simulink model "ElectronicStabilityControl"  (R2025b)
settings: configuration reference "VehicleFixed10ms" (kept outside this file)
undefined symbols (not defined in the file): CtrlBcuTrlrBrkGain, PlntVehDstCGFrntAxl, PlntVehDstCGRearAxl, vehdynicon
libraries: slpidlib x1, simulink x1
settings Model: DataDictionary=VirtualVehicleTemplate.sldd  ModifiedByFormat=The MathWorks, Inc.  Creator=The MathWorks, Inc.  LastModifiedBy=The MathWorks, Inc.
settings ConfigSetRef: SourceName=VehicleFixed10ms

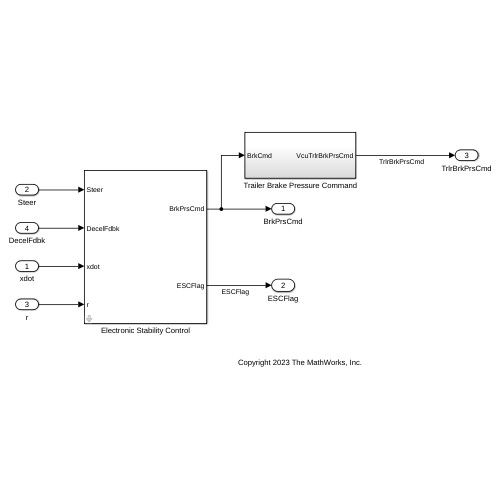
[thumbnail: Simulink's stored preview of the top-level diagram]
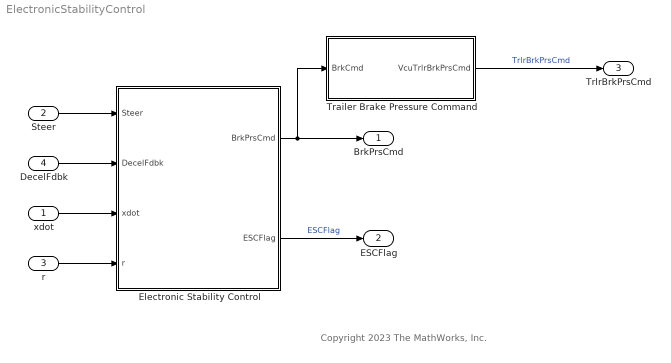
== system ElectronicStabilityControl ==
  note: Copyright 2023 The MathWorks, Inc.
  xdot : Inport  OutDataTypeStr=double  PortDimensions=1
  Steer : Inport  Port=2  OutDataTypeStr=double  PortDimensions=1
  r : Inport  Port=3  OutDataTypeStr=double  PortDimensions=1
  DecelFdbk : Inport  Port=4  OutDataTypeStr=double  PortDimensions=1
  Electronic Stability Control : Subsystem  mask{USG=1.15, xdot_en=2, L=PlntVehDstCGFrntAxl + PlntVehDstCGRearAxl, g=9.8, mu=1, xdotbpt=[-60:10:60], PGain=[.1 .2 .5 .8 1.5 3.0 0 3.0 1.5 .8 .5 .2 .1]}
      mask prompts: USG "Understeering gradient, USG [deg/g]:"; xdot_en "Speed threshold of ESC activation, xdot_en [m/s]:"; L "Wheel base, L [m]:"; g "Gravity acceleration, g [m/s^2]:"; mu "Tire-road scaling friction coefficient, mu []:"; xdotbpt "Speed breakpoints, xdotbpt [m/s]:"; PGain "P gain table data, PGain []:"
      mask help: This block offers Electronic Stability Control (ESC), a system designed to uphold a vehicle lateral and yaw stability by autonomously modulating brake pressure.
      mask init:
      | vehdynicon('vehdynalgo', gcb);
      mask DialogControl Container4 Prompt: Constants
      mask DialogControl Container3 Prompt: Controller parameters
  Trailer Brake Pressure Command : Subsystem
  BrkPrsCmd : Outport  OutDataTypeStr=double  VectorParamsAs1DForOutWhenUnconnected=off
  ESCFlag : Outport  Port=2  OutDataTypeStr=boolean
  TrlrBrkPrsCmd : Outport  Port=3  PortDimensions=6  VectorParamsAs1DForOutWhenUnconnected=off
  wires:
  Trailer Brake Pressure Command/1(VcuTrlrBrkPrsCmd) -> TrlrBrkPrsCmd/1  "TrlrBrkPrsCmd"
  Electronic Stability Control/1(BrkPrsCmd) -> Trailer Brake Pressure Command/1(BrkCmd), BrkPrsCmd/1
  Electronic Stability Control/2(ESCFlag) -> ESCFlag/1  "ESCFlag"
  xdot/1 -> Electronic Stability Control/3(xdot)
  r/1 -> Electronic Stability Control/4(r)
  DecelFdbk/1 -> Electronic Stability Control/2(DecelFdbk)
  Steer/1 -> Electronic Stability Control/1(Steer)

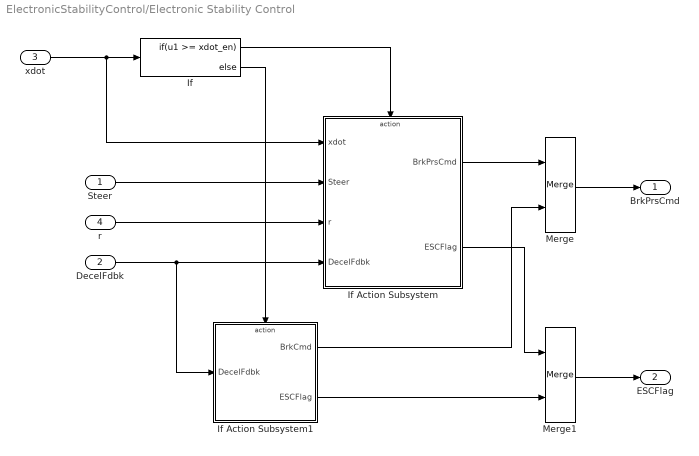
== system ElectronicStabilityControl/Electronic Stability Control ==
  Steer : Inport
  DecelFdbk : Inport  Port=2
  xdot : Inport  Port=3
  r : Inport  Port=4
  If : If  IfExpression=u1 >= xdot_en
  If Action Subsystem : Subsystem  TreatAsAtomicUnit=on
  If Action Subsystem1 : Subsystem  TreatAsAtomicUnit=on
  Merge : Merge
  Merge1 : Merge
  BrkPrsCmd : Outport
  ESCFlag : Outport  Port=2
  wires:
  xdot/1 -> If Action Subsystem/1(xdot), If/1
  Steer/1 -> If Action Subsystem/2(Steer)
  r/1 -> If Action Subsystem/3(r)
  Merge/1 -> BrkPrsCmd/1
  Merge1/1 -> ESCFlag/1
  If/1 -> If Action Subsystem/Action
  DecelFdbk/1 -> If Action Subsystem1/1(DecelFdbk), If Action Subsystem/4(DecelFdbk)
  If/2 -> If Action Subsystem1/Action
  If Action Subsystem1/1(BrkCmd) -> Merge/2
  If Action Subsystem1/2(ESCFlag) -> Merge1/2
  If Action Subsystem/2(ESCFlag) -> Merge1/1
  If Action Subsystem/1(BrkPrsCmd) -> Merge/1

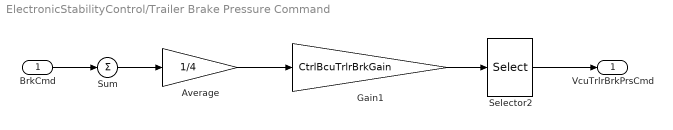
== system ElectronicStabilityControl/Trailer Brake Pressure Command ==
  BrkCmd : Inport
  Average : Gain  Gain=1/4
  Gain1 : Gain  Gain=CtrlBcuTrlrBrkGain
  Selector2 : Selector  InputPortWidth=1  IndexOptions=Index vector (dialog)  Indices=[1 1 1 1 1 1]  OutputSizes=1
  Sum : Sum  Inputs=+
  VcuTrlrBrkPrsCmd : Outport
  wires:
  Gain1/1 -> Selector2/1
  Average/1 -> Gain1/1
  BrkCmd/1 -> Sum/1
  Sum/1 -> Average/1
  Selector2/1 -> VcuTrlrBrkPrsCmd/1

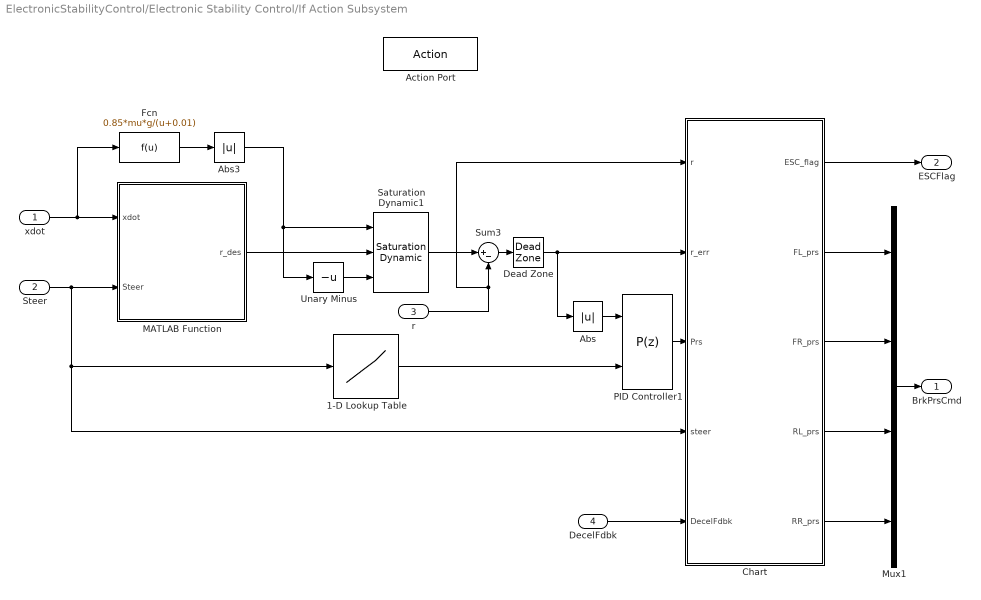
== system ElectronicStabilityControl/Electronic Stability Control/If Action Subsystem ==
  xdot : Inport
  Steer : Inport  Port=2
  r : Inport  Port=3
  DecelFdbk : Inport  Port=4
  Action Port : ActionPort
  1-D Lookup Table : Lookup_n-D  NumberOfTableDimensions=1  BreakpointsForDimension1=xdotbpt  Table=PGain  InternalRulePriority=Speed  RndMeth=Simplest
  Abs : Abs  SaturateOnIntegerOverflow=off
  Abs3 : Abs  SaturateOnIntegerOverflow=off
  Chart : Stateflow chart  InitFcn=vehdynicon('vehdynalgo', gcb);  TreatAsAtomicUnit=on
  Dead Zone : DeadZone  LowerValue=-0.001  UpperValue=0.001
  Fcn : Fcn  Expr=0.85*mu*g/(u+0.01)
  MATLAB Function : MATLAB Function  InitFcn=vehdynicon('vehdynalgo', gcb);  TreatAsAtomicUnit=on
  Mux1 : Mux
  PID Controller1 : slpidlib/PID Controller  Controller=P  Form=Parallel  TimeDomain=Discrete-time  UseExternalTs=off  SampleTime=-1  IntegratorMethod=Forward Euler  FilterMethod=Forward Euler  ControllerParametersSource=external  P=1  I=1  UseKiTs=off  D=0  UseExternalDerivativeSource=off  N=100  UseFilter=on  TunerSelectOption=Transfer Function Based (PID Tuner App)  ZeroCross=off  InitialConditionSource=internal  InitialConditionForIntegrator=0  InitialConditionForFilter=0  DifferentiatorICPrevScaledInput=0  ExternalReset=none  TrackingMode=off  Kt=1  LimitOutput=on  SatLimitsSource=internal  UpperSaturationLimit=1  LowerSaturationLimit=0  LinearizeAsGain=on  AntiWindupMode=none  Kb=1  LimitIntegrator=off  UpperIntegratorSaturationLimit=inf  LowerIntegratorSaturationLimit=-inf  POutMin=[]  POutMax=[]  IOutMin=[]  IOutMax=[]  DOutMin=[]  DOutMax=[]  NOutMin=[]  NOutMax=[]  SumOutMin=[]  SumOutMax=[]  SaturationOutMin=[]  SaturationOutMax=[]  PParamMin=[]  PParamMax=[]  IParamMin=[]  IParamMax=[]  DParamMin=[]  DParamMax=[]  NParamMin=[]  NParamMax=[]  KbParamMin=[]  KbParamMax=[]  KtParamMin=[]  KtParamMax=[]  KbOutMin=[]  KbOutMax=[]  KtOutMin=[]  KtOutMax=[]  IntegratorOutMin=[]  IntegratorOutMax=[]  FilterOutMin=[]  FilterOutMax=[]  SumI1OutMin=[]  SumI1OutMax=[]  SumI2OutMin=[]  SumI2OutMax=[]  SumI3OutMin=[]  SumI3OutMax=[]  SumI4OutMin=[]  SumI4OutMax=[]  SumDOutMin=[]  SumDOutMax=[]  DifferentiatorOutMin=[]  DifferentiatorOutMax=[]  FilterDiffOutCoefMin=[]  FilterDiffOutCoefMax=[]  ReciprocalOutMin=[]  ReciprocalOutMax=[]  SumDenOutMin=[]  SumDenOutMax=[]  SumNumOutMin=[]  SumNumOutMax=[]  DivideOutMin=[]  DivideOutMax=[]  UdiffTsProdOutMin=[]  UdiffTsProdOutMax=[]  NTsProdOutMin=[]  NTsProdOutMax=[]  UintegralTsProdOutMin=[]  UintegralTsProdOutMax=[]  UngainTsProdOutMin=[]  UngainTsProdOutMax=[]  ClampingZeroOutDataTypeStr=Inherit: Inherit via back propagation  ClampingZeroOutMin=[]  ClampingZeroOutMax=[]  FilterDenConstantOutDataTypeStr=Inherit: Inherit via back propagation  FilterDenConstantOutMin=[]  FilterDenConstantOutMax=[]  PCopyOutDataTypeStr=Inherit: Inherit via back propagation  PCopyOutMin=[]  PCopyOutMax=[]  NCopyOutDataTypeStr=Inherit: Inherit via back propagation  NCopyOutMin=[]  NCopyOutMax=[]  IntegratorContinuousStateAttributes=''  IntegratorStateMustResolveToSignalObject=off  IntegratorRTWStateStorageClass=Auto  FilterContinuousStateAttributes=''  FilterStateMustResolveToSignalObject=off  FilterRTWStateStorageClass=Auto  ParallelPVariant=ExternalParameters  IdealPVariant=Disabled  IVariant=Disabled  DVariant=Disabled  IntegratorVariant=Disabled  SatVariant=Enabled  AWVariant=Disabled  PCopyVariant=Disabled  TRVariant=Disabled  FdbkBlocksVariant=Forward  IdealPFdbkVariant=Disabled  SatFdbkVariant=Disabled  DerivativeFilterVariant=Disabled  NVariant=Disabled  NCopyVariant=Disabled_SignalSpec  FilterICVariant=Disabled  IntegratorICVariant=Disabled  ExternalResetVariant=Disabled  TRSumVariant=Passthrough  SumFdbkVariant=Disabled  SumVariant=Passthrough_P  TsampFilterVariant=InternalTs  TsampNgainVariant=Passthrough  TsampIntegralVariant=Disabled_SignalSpec  ExternalSaturationOutDataTypeStr=Inherit: Same as second input  DerivativeSourceVariant=Disabled  PreIntVariant=InternalPreInt
  Saturation Dynamic1 : simulink/Discontinuities/Saturation Dynamic  OutMin=[]  OutMax=[]  OutDataTypeStr=Inherit: Same as second input  OutDataType=fixdt(1, 16)  OutScaling=2^-10  DoSatur=off
  Sum3 : Sum  Inputs=|+-
  Unary Minus : UnaryMinus
  BrkPrsCmd : Outport
  ESCFlag : Outport  Port=2
  wires:
  MATLAB Function/1(r_des) -> Saturation Dynamic1/2
  Chart/4(RL_prs) -> Mux1/3
  Fcn/1 -> Abs3/1
  Mux1/1 -> BrkPrsCmd/1
  Unary Minus/1 -> Saturation Dynamic1/3
  Chart/1(ESC_flag) -> ESCFlag/1
  Chart/3(FR_prs) -> Mux1/2
  Chart/2(FL_prs) -> Mux1/1
  xdot/1 -> Fcn/1, MATLAB Function/1(xdot)
  Sum3/1 -> Dead Zone/1
  Abs3/1 -> Unary Minus/1, Saturation Dynamic1/1
  PID Controller1/1 -> Chart/3(Prs)
  1-D Lookup Table/1 -> PID Controller1/2
  r/1 -> Sum3/2, Chart/1(r)
  Steer/1 -> Chart/4(steer), 1-D Lookup Table/1, MATLAB Function/2(Steer)
  Dead Zone/1 -> Chart/2(r_err), Abs/1
  Saturation Dynamic1/1 -> Sum3/1
  Chart/5(RR_prs) -> Mux1/4
  DecelFdbk/1 -> Chart/5(DecelFdbk)
  Abs/1 -> PID Controller1/1

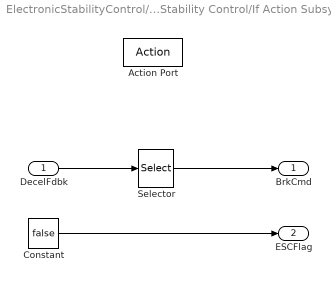
== system ElectronicStabilityControl/Electronic Stability Control/If Action Subsystem1 ==
  DecelFdbk : Inport
  Action Port : ActionPort
  Constant : Constant  Value=false
  Selector : Selector  InputPortWidth=1  IndexOptions=Index vector (dialog)  Indices=[1 1 1 1]  OutputSizes=1
  BrkCmd : Outport
  ESCFlag : Outport  Port=2
  wires:
  DecelFdbk/1 -> Selector/1
  Selector/1 -> BrkCmd/1
  Constant/1 -> ESCFlag/1

== stateflow chart ElectronicStabilityControl/Electronic Stability Control/If Action Subsystem/Chart ==
  state FrntLft_Brake
    entry, during:
    ESC_flag = true;
    FL_prs = Prs;
    FR_prs = 0;
    RL_prs = 0;
    RR_prs = 0;
  state Ready
    entry, during:
    ESC_flag = false;
    FL_prs = DecelFdbk;
    FR_prs = DecelFdbk;
    RL_prs = DecelFdbk;
    RR_prs = DecelFdbk;
  state FrntRght_Brake
    entry, during:
    ESC_flag = true;
    FL_prs = 0;
    FR_prs = Prs;
    RL_prs = 0;
    RR_prs = 0;
  state Entrance
    entry, during:
    ESC_flag = false;
    FL_prs = DecelFdbk;
    FR_prs = DecelFdbk;
    RL_prs = DecelFdbk;
    RR_prs = DecelFdbk;
  state RearLft_Brake
    entry, during:
    ESC_flag = true;
    FL_prs = 0;
    FR_prs = 0;
    RL_prs = Prs;
    RR_prs = 0;
  state RearRght_Brake
    entry, during:
    ESC_flag = true;
    FL_prs = 0;
    FR_prs = 0;
    RL_prs = Prs;
    RR_prs = 0;
  Ready -> FrntLft_Brake [order 1] : [(r_err < -0.05) &&(abs(steer)<=0.01|| r >0)]
  FrntLft_Brake -> RearRght_Brake [order 2] : [steer < -0.01 && r < 0]
  FrntLft_Brake -> Ready [order 1] : [abs(r_err) < 0.05]
  (default) -> Entrance
  Ready -> FrntRght_Brake [order 2] : [(r_err > 0.05) &&(abs(steer)<=0.01|| r < 0)]
  Entrance -> Ready : [abs(r_err) > 0.05 && abs(steer) > 0.01]
  FrntRght_Brake -> RearLft_Brake [order 2] : [steer > 0.01 && r > 0]
  FrntRght_Brake -> Ready [order 1] : [abs(r_err) < 0.05]
  Ready -> Entrance [order 5] : [abs(r_err) <= 0.05 && abs(steer) <= 0.01]
  Ready -> RearLft_Brake [order 3] : [r < 0 && r_err <-0.05]
  RearLft_Brake -> Ready : [abs(r_err) < 0.05]
  Ready -> RearRght_Brake [order 4] : [r > 0 && r_err > 0.05]
  RearRght_Brake -> Ready : [abs(r_err) < 0.05]
  data: ESC_flag output; FL_prs output; FR_prs output; RL_prs output; RR_prs output; r input; r_err input; Prs input; steer input; DecelFdbk input

== matlab function ElectronicStabilityControl/Electronic Stability Control/If Action Subsystem/MATLAB Function ==
  data: xdot input; Steer input; r_des output; USG parameter; L parameter; g parameter
function r_des = fcn(xdot, Steer, USG, L, g)

r_des = xdot*Steer/(L+USG*xdot^2/(57.3*g));
